simulink model "ISReferenceApplication"  (R2024b)
settings: Solver=ode4  StartTime=0.0  StopTime=60  FixedStep=1e-3  RelTol=5e-2
model workspace (MAT data in the model file):
  Downshift_Speeds = [9.5625  23.0625  36.5625  47.8125  59.0625  68.90625  78.75; 12.9375  26.4375  39.9375  51.1875  62.4375  72.84375  83.25; 16.3125  29.8125  43.3125  54.5625  65.8125  76.78125  87.75; 19.6875  33.1875  46.6875  57.9375  69.1875  80.71875  92.25]
  EngRevLim = 7000
  Pedal_Positions = [0.1 0.4 0.5 0.9]
  Upshift_Speeds = [12.9375  26.4375  39.9375  51.1875  62.4375  72.84375  83.25; 16.3125  29.8125  43.3125  54.5625  65.8125  76.78125  87.75; 19.6875  33.1875  46.6875  57.9375  69.1875  80.71875  92.25; 33  52.5  77.25  100.5  138.75  161.875  185]
  VEH.Mass = 1181
  VEH.StaticNormalFrontLoad.FR = 264.666666667
  VEH.StaticNormalFrontLoad.FL = 264.666666667
  VEH.StaticNormalRearLoad.RR = 322
  VEH.StaticNormalRearLoad.RL = 322
  VEH.WheelBase = 3.075
  VEH.FrontAxlePositionfromCG = 1.515
  VEH.RearAxlePositionfromCG = 1.504
  VEH.HeightCG = 0.134
  VEH.FrontalArea = 2.11
  VEH.DragCoefficient = 0.33
  VEH.NumberOfWheelsPerAxle = 2
  VEH.PitchMomentInertia = 1922.66666667
  VEH.RollMomentInertia = 432.333333333
  VEH.YawMomentInertia = 2066
  VEH.SteeringRatio = 18
  VEH.TrackWidth = 1.922
  VEH.SprungMass = 1096.72266667
  VEH.InitialLongPosition = 0
  VEH.InitialLatPosition = 0
  VEH.InitialVertPosition = 0
  VEH.InitialRollAngle = 0
  VEH.InitialPitchAngle = 0
  VEH.InitialYawAngle = 0
  VEH.InitialLongVel = 0
  VEH.InitialLatVel = 0
  VEH.InitialVertVel = 0
  VEH.InitialRollRate = 0
  VEH.InitialPitchRate = 0
  VEH.InitialYawRate = 0
  VEH.UnsprungMassRearAxle = 160
  VEH.UnsprungMassFrontAxle = 100
  rayDirections = [0  0  -1; 0  0  -1; 0  0  -1; 0  0  -1; 0  0  -1; 0  0  -1; 0  0  -1; 0  0  -1; 0  0  -1; 0  0  -1; 0  0  -1; 0  0  -1; 0  0  -1; 0  0  -1; 0  0  -1; 0  0  -1; 0  0  -1; 0  0  -1; 0  0  -1; 0  0  -1; 0  0  -1; 0  0  -1; 0  0  -1; 0  0  -1; 0  0  -1; 0  0  -1; 0  0  -1; 0  0  -1; 0  0  -1; 0  0  -1; 0  0  -1; 0  0  -1; 0  0  -1; 0  0  -1; 0  0  -1; 0  0  -1; 0  0  -1; 0  0  -1; 0  0  -1; 0  0  -1; 0  0  -1; 0  0  -1; 0  0  -1; 0  0  -1; 0  0  -1; 0  0  -1; 0  0  -1; 0  0  -1; 0  0  -1; 0  0  -1; 0  0  -1; 0  0  -1; 0  0  -1; 0  0  -1; 0  0  -1; 0  0  -1; 0  0  -1; 0  0  -1; 0  0  -1; 0  0  -1; 0  0  -1; 0  0  -1; 0  0  -1; 0  0  -1; 0  0  -1; 0  0  -1; 0  0  -1; 0  0  -1; 0  0  -1; 0  0  -1; 0  0  -1; 0  0  -1; 0  0  -1; 0  0  -1; 0  0  -1; 0  0  -1; 0  0  -1; 0  0  -1; 0  0  -1; 0  0  -1; 0  0  -1; 0  0  -1; 0  0  -1; 0  0  -1; 0  0  -1; 0  0  -1; 0  0  -1; 0  0  -1; 0  0  -1; 0  0  -1; 0  0  -1; 0  0  -1; 0  0  -1; 0  0  -1; 0  0  -1; 0  0  -1; 0  0  -1; 0  0  -1; 0  0  -1; 0  0  -1; 0  0  -1; 0  0  -1; 0  0  -1; 0  0  -1; 0  0  -1; 0  0  -1; 0  0  -1; 0  0  -1; 0  0  -1; 0  0  -1; 0  0  -1; 0  0  -1; 0  0  -1; 0  0  -1; 0  0  -1; 0  0  -1; 0  0  -1; 0  0  -1; 0  0  -1; 0  0  -1; 0  0  -1]
  rayLengths = [20; 20; 20; 20; 20; 20; 20; 20; 20; 20; 20; 20; 20; 20; 20; 20; 20; 20; 20; 20; 20; 20; 20; 20; 20; 20; 20; 20; 20; 20; 20; 20; 20; 20; 20; 20; 20; 20; 20; 20; 20; 20; 20; 20; 20; 20; 20; 20; 20; 20; 20; 20; 20; 20; 20; 20; 20; 20; 20; 20; 20; 20; 20; 20; 20; 20; 20; 20; 20; 20; 20; 20; 20; 20; 20; 20; 20; 20; 20; 20; 20; 20; 20; 20; 20; 20; 20; 20; 20; 20; 20; 20; 20; 20; 20; 20; 20; 20; 20; 20; 20; 20; 20; 20; 20; 20; 20; 20; 20; 20; 20; 20; 20; 20; 20; 20; 20; 20; 20; 20; 20]
  rayOrigins = [0.5  -0.5  0; 0.4  -0.5  0; 0.3  -0.5  0; 0.2  -0.5  0; 0.1  -0.5  0; 0  -0.5  0; -0.1  -0.5  0; -0.2  -0.5  0; -0.3  -0.5  0; -0.4  -0.5  0; -0.5  -0.5  0; 0.5  -0.4  0; 0.4  -0.4  0; 0.3  -0.4  0; 0.2  -0.4  0; 0.1  -0.4  0; 0  -0.4  0; -0.1  -0.4  0; -0.2  -0.4  0; -0.3  -0.4  0; -0.4  -0.4  0; -0.5  -0.4  0; 0.5  -0.3  0; 0.4  -0.3  0; 0.3  -0.3  0; 0.2  -0.3  0; 0.1  -0.3  0; 0  -0.3  0; -0.1  -0.3  0; -0.2  -0.3  0; -0.3  -0.3  0; -0.4  -0.3  0; -0.5  -0.3  0; 0.5  -0.2  0; 0.4  -0.2  0; 0.3  -0.2  0; 0.2  -0.2  0; 0.1  -0.2  0; 0  -0.2  0; -0.1  -0.2  0; -0.2  -0.2  0; -0.3  -0.2  0; -0.4  -0.2  0; -0.5  -0.2  0; 0.5  -0.1  0; 0.4  -0.1  0; 0.3  -0.1  0; 0.2  -0.1  0; 0.1  -0.1  0; 0  -0.1  0; -0.1  -0.1  0; -0.2  -0.1  0; -0.3  -0.1  0; -0.4  -0.1  0; -0.5  -0.1  0; 0.5  0  0; 0.4  0  0; 0.3  0  0; 0.2  0  0; 0.1  0  0; 0  0  0; -0.1  0  0; -0.2  0  0; -0.3  0  0; -0.4  0  0; -0.5  0  0; 0.5  0.1  0; 0.4  0.1  0; 0.3  0.1  0; 0.2  0.1  0; 0.1  0.1  0; 0  0.1  0; -0.1  0.1  0; -0.2  0.1  0; -0.3  0.1  0; -0.4  0.1  0; -0.5  0.1  0; 0.5  0.2  0; 0.4  0.2  0; 0.3  0.2  0; 0.2  0.2  0; 0.1  0.2  0; 0  0.2  0; -0.1  0.2  0; -0.2  0.2  0; -0.3  0.2  0; -0.4  0.2  0; -0.5  0.2  0; 0.5  0.3  0; 0.4  0.3  0; 0.3  0.3  0; 0.2  0.3  0; 0.1  0.3  0; 0  0.3  0; -0.1  0.3  0; -0.2  0.3  0; -0.3  0.3  0; -0.4  0.3  0; -0.5  0.3  0; 0.5  0.4  0; 0.4  0.4  0; 0.3  0.4  0; 0.2  0.4  0; 0.1  0.4  0; 0  0.4  0; -0.1  0.4  0; -0.2  0.4  0; -0.3  0.4  0; -0.4  0.4  0; -0.5  0.4  0; 0.5  0.5  0; 0.4  0.5  0; 0.3  0.5  0; 0.2  0.5  0; 0.1  0.5  0; 0  0.5  0; -0.1  0.5  0; -0.2  0.5  0; -0.3  0.5  0; -0.4  0.5  0; -0.5  0.5  0]
  temp.Mass = 1181
  temp.StaticNormalFrontLoad.FR = 264.666666667
  temp.StaticNormalFrontLoad.FL = 264.666666667
  temp.StaticNormalRearLoad.RR = 322
  temp.StaticNormalRearLoad.RL = 322
  temp.WheelBase = 2.86
  temp.FrontAxlePositionfromCG = 1.43
  temp.RearAxlePositionfromCG = 1.43
  temp.HeightCG = 0.134
  temp.FrontalArea = 2.11
  temp.DragCoefficient = 0.33
  temp.NumberOfWheelsPerAxle = 2
  temp.PitchMomentInertia = 1922.66666667
  temp.RollMomentInertia = 432.333333333
  temp.YawMomentInertia = 2066
  temp.SteeringRatio = 18
  temp.TrackWidth = 1.485
  temp.SprungMass = 1096.72266667
  temp.InitialLongPosition = 590.01904884
  temp.InitialLatPosition = 11.2130507532
  temp.InitialVertPosition = -0.6630556109
  temp.InitialRollAngle = -0.0172848662
  temp.InitialPitchAngle = 0.0033932423
  temp.InitialYawAngle = 0.001924738
  temp.InitialLongVel = 0
  temp.InitialLatVel = 0
  temp.InitialVertVel = 0
  temp.InitialRollRate = 0
  temp.InitialPitchRate = 0
  temp.InitialYawRate = 0
  temp.UnsprungMassRearAxle = 160
  temp.UnsprungMassFrontAxle = 100
  temp.VehicleWidth = 1.731
  temp.VehicleLength = 4.769
  temp.diameter = 0.653
  temp.DrawFreq = 0.1
  temp.T_ref = [0 0.173579329608 0.347158660043 0.520737996807 0.69431733453 0.867896671781 1.04147600843 1.21505534588 1.38863468425 1.56221402051 1.73579335734 1.90937269505 ... (14403 elements, 4801x3)]
undefined symbols (not defined in the file): DiscIntNeverNeededParam, Sim3dSensor
libraries: simulink x14, autolibutils x7, slpidlib x2, vehdynlibviscommon x2, sim3dgroundtruthsensorlib x2, autolibtranscontrolscommon x1, autolibshared x1, vehdynlibdriver x1, sharedtransform x1, vehdynlibsens x1, vehdynlibscenariocommon x1, sim3dlib x1
(part 1 of 4)
settings Model: DataDictionary=ISReferenceApplication.sldd  ModifiedByFormat=The MathWorks, Inc.  SimulationMode=accelerator  Creator=The MathWorks, Inc.  LastModifiedBy=The MathWorks, Inc.
settings SolverCC: SolverJacobianMethodControl=FullPerturbation  ZeroCrossAlgorithm=Adaptive  AlgebraicLoopSolver=TrustRegion  DecoupledContinuousIntegration=on  MinimalZcImpactIntegration=on  MaxZcPerStep=1
settings DataIOCC: ReturnWorkspaceOutputs=off
settings OptimizationCC: ReuseModelBlockBuffer=off
settings DebuggingCC: SignalInfNanChecking=error  ArtificialAlgebraicLoopMsg=none  MaskedZcDiagnostic=none  IgnoredZcDiagnostic=none  UnconnectedInputMsg=warning  UnconnectedOutputMsg=warning  UnconnectedLineMsg=warning  PregeneratedLibrarySubsystemCodeDiagnostic=none  ArithmeticOperatorsInVariantConditions=warning
settings ModelReferenceCC: UpdateModelReferenceTargets=IfOutOfDate  EnableRefExpFcnMdlSchedulingChecks=on  ModelReferenceMinAlgLoopOccurrences=on  PropagateSignalLabelsOutOfModel=off
settings SFSimCC: SimUseLocalCustomCode=off
settings RTWCC: RTWUseLocalCustomCode=off  GPUComputeCapability=3.5  DLArmComputeVersion=19.05

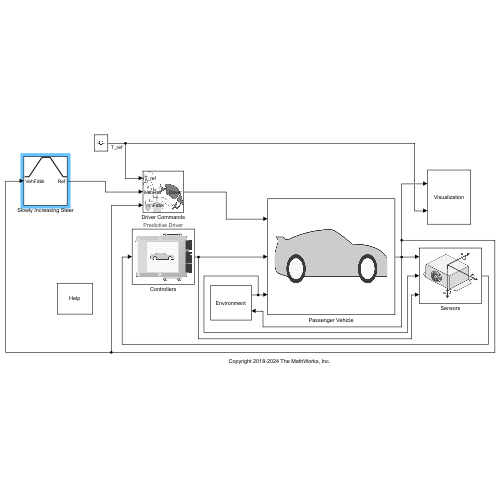
[thumbnail: Simulink's stored preview of the top-level diagram]
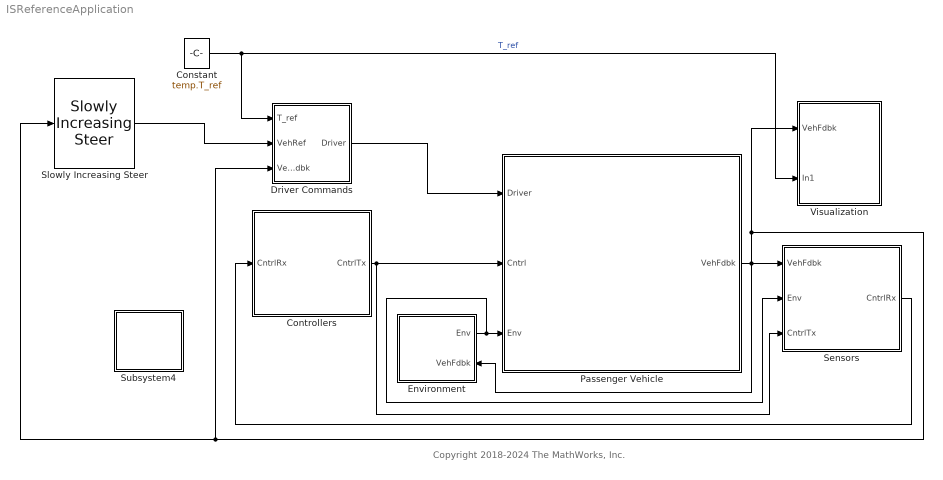
== system ISReferenceApplication ==
  note: Copyright 2018-2024 The MathWorks, Inc.
  Constant : Constant  Value=temp.T_ref  VectorParams1D=off
  Controllers : Subsystem
      mask Display: image('SystemControllers.png')
  Driver Commands : Subsystem  VariantControl=0  mask{driverType=Predictive Driver}
      mask prompts: driverType "Vehicle command mode"
      mask init:
      | [~]=vdynblksdrvrconfig(gcb)
      settings: AttributesFormatString=%<driverType>
      mask Help: eval('vdynblkshelp(''vdcrdriver'')');
      mask TypeOptions driverType: Longitudinal Driver | Predictive Driver | Open Loop
      mask Display: image('driverlatlong.png');
  Environment : Subsystem
      settings: PortSchema="{\"entries\":[{\"content\":{\"sides\":[{\"content\":{\"connectorIds\":[]},\"type\":\"ConnectorPlacement.EquallySpacedRectSide\",\"uuid\":\"7e477c5b-2979-4b31-83f8-8e06b5171f31\"},{\"content\":{\"connectorIds\":[\"Out1\",\"In1\"],\"side\":\"RIGHT\"},\"type\":\"ConnectorPlacement.EquallySpacedRectSide\",\"uuid\":\"d70ab29f-7073-466b-949c-fd6d019fdbd7\"},{\"content\":{\"connectorIds\":[],\"side\":\"TOP\"},\"type\":\"ConnectorPlacement.EquallySpacedRectSide\",\"uuid\":\"2d86cca8-a415-4272-bacd-17a50325dd7c\"}]},\"type\":\"ConnectorPlacement.EquallySpacedConnector\",\"uuid\":\"3f48fc9c-531e-41c0-b546-1206e5799aa8\"}],\"packageUris\":[\"http://schema.mathworks.com/mf0/Connector/R2020b\"],\"version\":\"1.0\"}"
      mask Display: disp('Environment')
  Passenger Vehicle : Subsystem
      mask Display: image('PassengerVehicle.png')
  Sensors : Subsystem
      mask Display: image('sensorimu.png'); % Use "Edit Image" on toolstrip to change.
  Slowly Increasing Steer : vehdynlibscenariocommon/Slowly Increasing Steer  ssMode=Initialize from model  ssVar=logsout  t_start=0  xdot_r=40  xdotUnit=km/hr  omega_hw=10  theta_max=270  t_stop=2  ay_max=.5  steerDir=off  ay_stop=off  ssDefault=on  X_o=0  Y_o=0  psi_o=0  ssTol=0.0001  ssMaxTime=10  ssWSName=is50mph  aMode=2
  Subsystem4 : Subsystem
      settings: OpenFcn=eval('vdynblkshelp(''vdynblksincreasingsteering'')');
      mask Display: disp('Help')
  Visualization : Subsystem
      mask Display: disp('Visualization')
  wires:
  Controllers/1(CntrlTx) -> Sensors/3(CntrlTx), Passenger Vehicle/2(Cntrl)
  Slowly Increasing Steer/1 -> Driver Commands/2(VehRef)
  Driver Commands/1(Driver) -> Passenger Vehicle/1(Driver)
  Sensors/1(CntrlRx) -> Controllers/1(CntrlRx)
  Environment/1(Env) -> Passenger Vehicle/3(Env), Sensors/2(Env)
  Passenger Vehicle/1(VehFdbk) -> Environment/1(VehFdbk), Sensors/1(VehFdbk), Visualization/1(VehFdbk), Driver Commands/3(VehFdbk), Slowly Increasing Steer/1
  Constant/1 -> Driver Commands/1(T_ref), Visualization/2(In1)  "T_ref"

== system ISReferenceApplication/Controllers ==
  CntrlRx : Inport
  Active Differential Control : Subsystem  Variant=on  VariantControlMode=label  LabelModeActiveChoice=0
  Brake Pressure Control : Subsystem  Variant=on  VariantControlMode=label  LabelModeActiveChoice=0
  Bus Creator : BusCreator  Inputs=1
  Bus Creator1 : BusCreator  Inputs=1
  Bus Creator2 : BusCreator  Inputs=3
  Bus Creator3 : BusCreator  Inputs=4
  Bus Creator4 : BusCreator  Inputs=1
  Bus Selector : BusSelector  OutputSignals=Driver.DecelFdbk,Wheels.Omega,IMU.Acc,Driver.AccFdbk,Wheels.BrkPrs
  Bus Selector1 : BusSelector  OutputSignals=Driver.AccFdbk,Driver.DecelFdbk,Driver.GearFdbk,Engine.EngSpd,Wheels.Omega
  Bus Selector2 : BusSelector  OutputSignals=Driver.AccFdbk,Engine.EngSpd
  Bus Selector3 : BusSelector  OutputSignals=Driver.AccFdbk,Driver.DecelFdbk,Driver.SteerFdbk,Driver.GearFdbk,Wheels.Omega,IMU.Acc,IMU.pqr
  ECU : Subsystem  SystemSampleTime=.01
  Ground : Ground
  Transmission Controller : Subsystem  Variant=on  VariantControlMode=label  VariantControl=Variant1  LabelModeActiveChoice=3
  CntrlTx : Outport  VectorParamsAs1DForOutWhenUnconnected=off
  wires:
  Bus Selector2/1 -> ECU/2(<Accel>)  "<AccFdbk>"
  Bus Creator/1 -> Bus Creator3/1  "ECU"
  Bus Creator1/1 -> Bus Creator3/2  "Transmission"
  Bus Creator3/1 -> CntrlTx/1  "CntrlTx"
  Bus Creator4/1 -> Bus Creator3/4  "Diff"
  Active Differential Control/1(DiffPrsCmd) -> Bus Creator4/1  "DiffPrsCmd"
  Active Differential Control/2(TrqCmd) -> [DiffTrqCmd]
  ECU/1(EngTrqCmd) -> Bus Creator/1  "EngTrqCmd"
  Transmission Controller/1(" Gear") -> Bus Creator1/1  "GearCmd"
  [DiffTrqCmd] -> ECU/1(DiffTrqCmd)  "DiffTrqCmd"
  Ground/1 -> Transmission Controller/7(UpReq), Transmission Controller/8(DownReq)
  Bus Selector2/2 -> ECU/3(EngSpd)  "<EngSpd>"
  Bus Selector1/5 -> Transmission Controller/5(Omega)  "<Omega>"
  Bus Selector1/2 -> Transmission Controller/2(BrkCmd)  "<DecelFdbk>"
  Bus Selector1/3 -> Transmission Controller/3(GearReq)  "<GearFdbk>"
  Bus Selector1/4 -> Transmission Controller/4(EngSpd)  "<EngSpd>"
  Bus Selector1/1 -> Transmission Controller/1(Accel)  "<AccFdbk>"
  Bus Selector3/1 -> Active Differential Control/1(Accel)  "<AccFdbk>"
  Bus Selector3/2 -> Active Differential Control/2(BrkCmd)  "<DecelFdbk>"
  Bus Selector3/3 -> Active Differential Control/3(Steer)  "<SteerFdbk>"
  Bus Selector3/4 -> Active Differential Control/4(GearFdbk)  "<GearFdbk>"
  Bus Selector3/5 -> Active Differential Control/5(Omega)  "<Omega>"
  Bus Selector3/6 -> Active Differential Control/6(axayaz)  "<Acc>"
  Bus Selector3/7 -> Active Differential Control/7(pqr)  "<pqr>"
  Bus Selector/1 -> Brake Pressure Control/1(DecelFdbk)  "<DecelFdbk>"
  CntrlRx/1 -> Bus Selector3/1, Bus Selector/1, Bus Selector1/1, Bus Selector2/1
  Bus Selector/2 -> Brake Pressure Control/2(Omega)  "<Omega>"
  Bus Selector/3 -> Brake Pressure Control/3(Accel)  "<Acc>"
  Brake Pressure Control/2(BrkPrsCmd) -> Bus Creator2/2  "BrkPrsCmd"
  Bus Creator2/1 -> Bus Creator3/3  "Brake"
  Brake Pressure Control/1(ABSFlag) -> [ABSFlag], Bus Creator2/1  "ABSFlag"
  [ABSFlag] -> Transmission Controller/6(ABSFlag)
  [ABSFlag] -> ECU/4(ABSFlag)
  Bus Selector/4 -> Brake Pressure Control/4(AccelFdbk)  "<AccFdbk>"
  Bus Selector/5 -> Brake Pressure Control/5(BrkPrs)  "<BrkPrs>"
  Brake Pressure Control/3(TCSFlag) -> Bus Creator2/3  "TCSFlag"

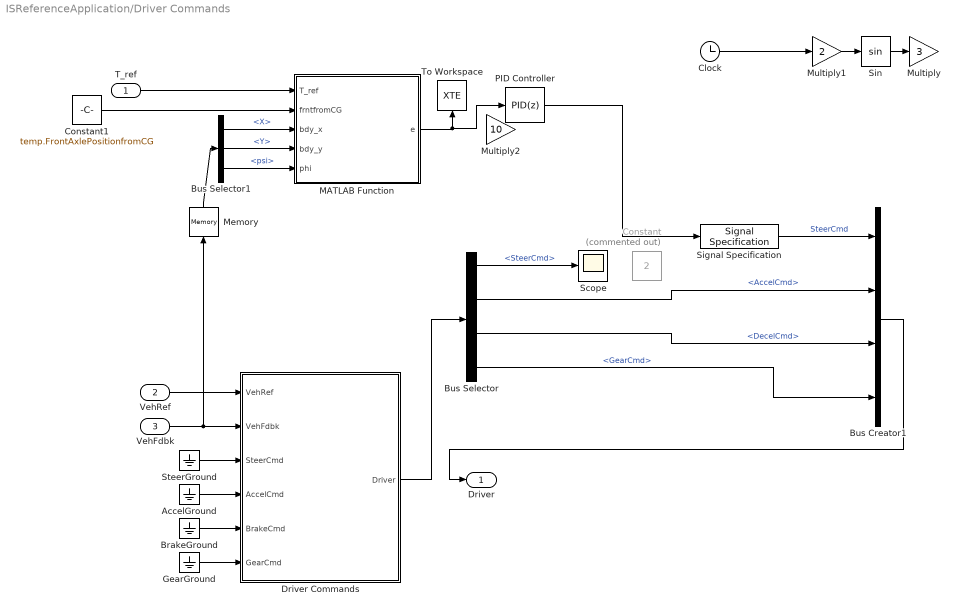
== system ISReferenceApplication/Driver Commands ==
  T_ref : Inport
  VehRef : Inport  Port=2
  VehFdbk : Inport  Port=3
  AccelGround : Ground
  BrakeGround : Ground
  Bus Creator1 : BusCreator  Inputs=4
  Bus Selector : BusSelector  OutputSignals=SteerCmd,AccelCmd,DecelCmd,GearCmd
  Bus Selector1 : BusSelector  OutputSignals=Body.InertFrm.Geom.Disp.X,Body.InertFrm.Geom.Disp.Y,Body.InertFrm.Cg.Ang.psi
  Clock : Clock
  Constant : Constant  Commented=on  Value=2
  Constant1 : Constant  Value=temp.FrontAxlePositionfromCG
  Driver Commands : Subsystem  Variant=on  VariantControl=Variant1  AllowZeroVariantControls=on
  GearGround : Ground
  MATLAB Function : MATLAB Function  TreatAsAtomicUnit=on
  Memory : Memory
  Multiply : Gain  Gain=3
  Multiply1 : Gain  Gain=2
  Multiply2 : Gain  Gain=10
  PID Controller : slpidlib/PID Controller  Controller=PID  Form=Parallel  TimeDomain=Discrete-time  UseExternalTs=off  SampleTime=-1  IntegratorMethod=Forward Euler  FilterMethod=Forward Euler  ControllerParametersSource=internal  P=10  I=10  UseKiTs=off  D=5  UseExternalDerivativeSource=off  N=100  UseFilter=on  TunerSelectOption=Transfer Function Based (PID Tuner App)  InitialConditionSource=internal  InitialConditionForIntegrator=0  InitialConditionForFilter=0  DifferentiatorICPrevScaledInput=0  ExternalReset=none  TrackingMode=off  Kt=1  LimitOutput=off  SatLimitsSource=internal  UpperSaturationLimit=inf  LowerSaturationLimit=-inf  LinearizeAsGain=on  AntiWindupMode=none  Kb=1  LimitIntegrator=off  UpperIntegratorSaturationLimit=inf  LowerIntegratorSaturationLimit=-inf  POutMin=[]  POutMax=[]  IOutMin=[]  IOutMax=[]  DOutMin=[]  DOutMax=[]  NOutMin=[]  NOutMax=[]  SumOutMin=[]  SumOutMax=[]  SaturationOutMin=[]  SaturationOutMax=[]  PParamMin=[]  PParamMax=[]  IParamMin=[]  IParamMax=[]  DParamMin=[]  DParamMax=[]  NParamMin=[]  NParamMax=[]  KbParamMin=[]  KbParamMax=[]  KtParamMin=[]  KtParamMax=[]  KbOutMin=[]  KbOutMax=[]  KtOutMin=[]  KtOutMax=[]  IntegratorOutMin=[]  IntegratorOutMax=[]  FilterOutMin=[]  FilterOutMax=[]  SumI1OutMin=[]  SumI1OutMax=[]  SumI2OutMin=[]  SumI2OutMax=[]  SumI3OutMin=[]  SumI3OutMax=[]  SumI4OutMin=[]  SumI4OutMax=[]  SumDOutMin=[]  SumDOutMax=[]  DifferentiatorOutMin=[]  DifferentiatorOutMax=[]  FilterDiffOutCoefMin=[]  FilterDiffOutCoefMax=[]  ReciprocalOutMin=[]  ReciprocalOutMax=[]  SumDenOutMin=[]  SumDenOutMax=[]  SumNumOutMin=[]  SumNumOutMax=[]  DivideOutMin=[]  DivideOutMax=[]  UdiffTsProdOutMin=[]  UdiffTsProdOutMax=[]  NTsProdOutMin=[]  NTsProdOutMax=[]  UintegralTsProdOutMin=[]  UintegralTsProdOutMax=[]  UngainTsProdOutMin=[]  UngainTsProdOutMax=[]  ClampingZeroOutDataTypeStr=Inherit: Inherit via back propagation  ClampingZeroOutMin=[]  ClampingZeroOutMax=[]  FilterDenConstantOutDataTypeStr=Inherit: Inherit via back propagation  FilterDenConstantOutMin=[]  FilterDenConstantOutMax=[]  PCopyOutDataTypeStr=Inherit: Inherit via back propagation  PCopyOutMin=[]  PCopyOutMax=[]  NCopyOutDataTypeStr=Inherit: Inherit via back propagation  NCopyOutMin=[]  NCopyOutMax=[]  IntegratorContinuousStateAttributes=''  IntegratorStateMustResolveToSignalObject=off  IntegratorRTWStateStorageClass=Auto  FilterContinuousStateAttributes=''  FilterStateMustResolveToSignalObject=off  FilterRTWStateStorageClass=Auto  ParallelPVariant=InternalParameters  IdealPVariant=Disabled  IVariant=InternalParameters  DVariant=InternalParameters  IntegratorVariant=Discrete  SatVariant=Disabled  AWVariant=Passthrough  PCopyVariant=Disabled  TRVariant=Disabled  FdbkBlocksVariant=Forward  IdealPFdbkVariant=Disabled  SatFdbkVariant=Disabled  DerivativeFilterVariant=ForwardEulerFilter  NVariant=InternalParameters  NCopyVariant=Disabled  FilterICVariant=InternalICsFilter  IntegratorICVariant=InternalICs  ExternalResetVariant=Disabled  TRSumVariant=Passthrough  SumFdbkVariant=Disabled  SumVariant=Sum_PID  TsampFilterVariant=InternalTs  TsampNgainVariant=Passthrough  TsampIntegralVariant=Disabled_SignalSpec  ExternalSaturationOutDataTypeStr=Inherit: Same as second input  DerivativeSourceVariant=ErrorSignal  PreIntVariant=InternalPreInt
  Scope : Scope
  Signal Specification : SignalSpecification  Unit=rad
  Sin : Trigonometry
  SteerGround : Ground
  To Workspace : ToWorkspace  VariableName=XTE  SaveFormat=Timeseries  SampleTime=-1
  Driver : Outport  VectorParamsAs1DForOutWhenUnconnected=off
  wires:
  VehRef/1 -> Driver Commands/1(VehRef)
  VehFdbk/1 -> Memory/1, Driver Commands/2(VehFdbk)
  Driver Commands/1(" Driver") -> Bus Selector/1
  SteerGround/1 -> Driver Commands/3(SteerCmd)
  AccelGround/1 -> Driver Commands/4(AccelCmd)
  BrakeGround/1 -> Driver Commands/5(BrakeCmd)
  GearGround/1 -> Driver Commands/6(GearCmd)
  Bus Selector/2 -> Bus Creator1/2  "<AccelCmd>"
  Bus Selector/3 -> Bus Creator1/3  "<DecelCmd>"
  Bus Selector/4 -> Bus Creator1/4  "<GearCmd>"
  Bus Selector/1 -> Scope/1  "<SteerCmd>"
  Signal Specification/1 -> Bus Creator1/1  "SteerCmd"
  Bus Creator1/1 -> Driver/1
  Clock/1 -> Multiply1/1
  Sin/1 -> Multiply/1
  Multiply1/1 -> Sin/1
  T_ref/1 -> MATLAB Function/1(T_ref)
  Bus Selector1/1 -> MATLAB Function/3(bdy_x)  "<X>"
  Bus Selector1/2 -> MATLAB Function/4(bdy_y)  "<Y>"
  Bus Selector1/3 -> MATLAB Function/5(phi)  "<psi>"
  MATLAB Function/1(e) -> PID Controller/1, To Workspace/1
  Memory/1 -> Bus Selector1/1
  Constant1/1 -> MATLAB Function/2(frntfromCG)
  PID Controller/1 -> Signal Specification/1

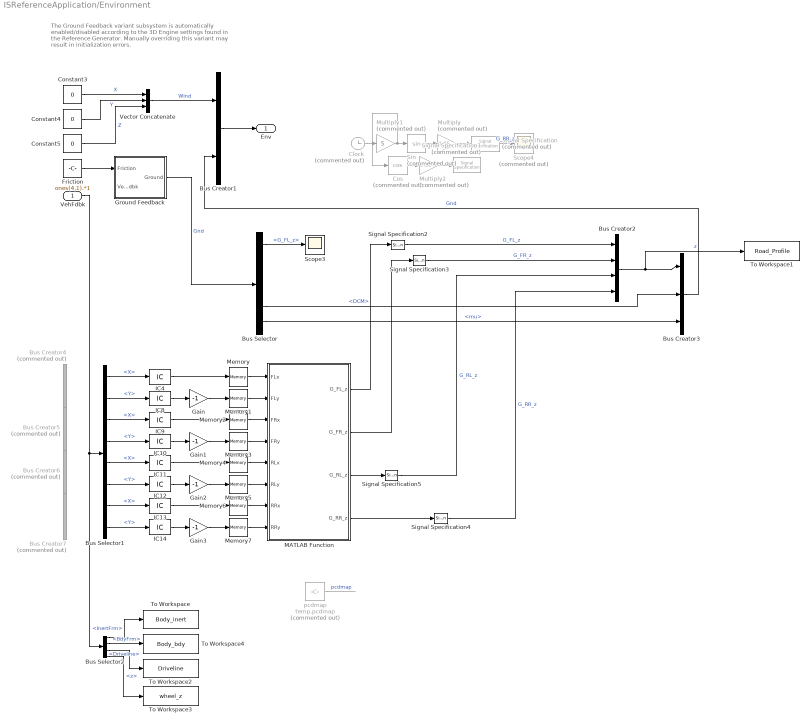
== system ISReferenceApplication/Environment ==
  note: The Ground Feedback variant subsystem is automatically enabled/disabled according to the 3D Engine settings found in the Reference Generator.
      | Manually overriding this variant may result in initialization errors.
  VehFdbk : Inport
  Bus Creator1 : BusCreator  Inputs=2
  Bus Creator2 : BusCreator  Inputs=4
  Bus Creator3 : BusCreator  Inputs=3
  Bus Creator{4..7} (4 alike) : BusCreator  Commented=on  Inputs=2
  Bus Selector : BusSelector  OutputSignals=z.G_FL_z,z.G_FR_z,z.G_RL_z,z.G_RR_z,DCM,mu
  Bus Selector1 : BusSelector  OutputSignals=Body.InertFrm.FrntAxl.Lft.Disp.X,Body.InertFrm.FrntAxl.Lft.Disp.Y,Body.InertFrm.FrntAxl.Rght.Disp.X,Body.InertFrm.FrntAxl.Rght.Disp.Y,Body.InertFrm.RearAxl.Lft.Disp.X,Body.InertFrm.RearAxl.Lft.Disp.Y,Body.InertFrm.RearAxl.Rght.Disp.X,Body.InertFrm.RearAxl.Rght.Disp.Y
  Bus Selector2 : BusSelector  OutputSignals=Body.InertFrm,Body.BdyFrm,Driveline,Wheels.TireFrame.z
  Clock : Clock  Commented=on
  Constant3 : Constant  Value=0
  Constant4 : Constant  Value=0
  Constant5 : Constant  Value=0
  Cos : Trigonometry  Commented=on  Operator=cos
  Friction : Constant  Value=ones(4,1).*1
  Gain{,1..3} (4 alike) : Gain  Gain=-1
  Ground Feedback : Subsystem  Variant=on  VariantControlMode=label  LabelModeActiveChoice=0
  IC{4,8..14} (8 alike) : InitialCondition  Value=0
  MATLAB Function : MATLAB Function  TreatAsAtomicUnit=on
  Memory : Memory  InitialCondition=temp.InitialLongPosition+temp.FrontAxlePositionfromCG  InheritSampleTime=on
  Memory1 : Memory  InitialCondition=-temp.InitialLatPosition-temp.TrackWidth  InheritSampleTime=on
  Memory2 : Memory  InitialCondition=temp.InitialLongPosition+temp.FrontAxlePositionfromCG  InheritSampleTime=on
  Memory3 : Memory  InitialCondition=-temp.InitialLatPosition+temp.TrackWidth  InheritSampleTime=on
  Memory4 : Memory  InitialCondition=temp.InitialLongPosition+temp.RearAxlePositionfromCG  InheritSampleTime=on
  Memory5 : Memory  InitialCondition=-temp.InitialLatPosition-temp.TrackWidth  InheritSampleTime=on
  Memory6 : Memory  InitialCondition=temp.InitialLongPosition+temp.RearAxlePositionfromCG  InheritSampleTime=on
  Memory7 : Memory  InitialCondition=-temp.InitialLatPosition+temp.TrackWidth  InheritSampleTime=on
  Multiply : Gain  Commented=on  Gain=0.05
  Multiply1 : Gain  Commented=on  Gain=5
  Multiply2 : Gain  Commented=on  Gain=0.05
  Scope3 : Scope
  Scope4 : Scope  Commented=on
  Signal Specification : SignalSpecification  Commented=on  Unit=m
  Signal Specification1 : SignalSpecification  Commented=on  Unit=m
  Signal Specification{2..5} (4 alike) : SignalSpecification  OutDataTypeStr=double  Unit=m
  Sin : Trigonometry  Commented=on
  To Workspace : ToWorkspace  VariableName=Body_inert  SaveFormat=Timeseries  SampleTime=-1
  To Workspace1 : ToWorkspace  VariableName=Road_Profile  SaveFormat=Timeseries  SampleTime=-1
  To Workspace2 : ToWorkspace  VariableName=Driveline  SaveFormat=Timeseries  SampleTime=-1
  To Workspace3 : ToWorkspace  VariableName=wheel_z  SaveFormat=Timeseries  SampleTime=-1
  To Workspace4 : ToWorkspace  VariableName=Body_bdy  SaveFormat=Timeseries  SampleTime=-1
  Vector Concatenate : Concatenate  NumInputs=3
  pcdmap : Constant  Commented=on  Value=temp.pcdmap
  Env : Outport  VectorParamsAs1DForOutWhenUnconnected=off
  wires:
  Constant5/1 -> Vector Concatenate/3  "Z"
  Vector Concatenate/1 -> Bus Creator1/1  "Wind"
  Constant3/1 -> Vector Concatenate/1  "X"
  Constant4/1 -> Vector Concatenate/2  "Y"
  Bus Creator1/1 -> Env/1
  Friction/1 -> Ground Feedback/1(Friction)
  VehFdbk/1 -> Bus Selector2/1, Bus Selector1/1
  Sin/1 -> Multiply/1
  Multiply/1 -> Signal Specification/1
  Signal Specification/1 -> Scope4/1  "G_RR_z"
  Bus Creator2/1 -> To Workspace1/1, Bus Creator3/1  "z"
  Bus Selector/5 -> Bus Creator3/2  "<DCM>"
  Bus Selector/6 -> Bus Creator3/3  "<mu>"
  Clock/1 -> Multiply1/1
  Multiply1/1 -> Cos/1, Sin/1
  Multiply2/1 -> Signal Specification1/1
  Cos/1 -> Multiply2/1
  Bus Selector/1 -> Scope3/1  "<G_FL_z>"
  pcdmap/1 -> ?  "pcdmap"
  Bus Selector1/1 -> IC4/1  "<X>"
  Bus Selector1/2 -> IC8/1  "<Y>"
  Bus Selector1/3 -> IC9/1  "<X>"
  Bus Selector1/4 -> IC10/1  "<Y>"
  Bus Selector1/5 -> IC11/1  "<X>"
  Bus Selector1/6 -> IC12/1  "<Y>"
  Bus Selector1/7 -> IC13/1  "<X>"
  Bus Selector1/8 -> IC14/1  "<Y>"
  IC4/1 -> Memory/1
  IC8/1 -> Gain/1
  IC9/1 -> Memory2/1
  IC10/1 -> Gain1/1
  IC11/1 -> Memory4/1
  IC12/1 -> Gain2/1
  IC13/1 -> Memory6/1
  IC14/1 -> Gain3/1
  Signal Specification2/1 -> Bus Creator2/1  "G_FL_z"
  Signal Specification3/1 -> Bus Creator2/2  "G_FR_z"
  Signal Specification4/1 -> Bus Creator2/4  "G_RR_z"
  Signal Specification5/1 -> Bus Creator2/3  "G_RL_z"
  MATLAB Function/1(G_FL_z) -> Signal Specification2/1
  MATLAB Function/2(G_FR_z) -> Signal Specification3/1
  MATLAB Function/3(G_RL_z) -> Signal Specification5/1
  MATLAB Function/4(G_RR_z) -> Signal Specification4/1
  Memory/1 -> MATLAB Function/1(FLx)
  Memory1/1 -> MATLAB Function/2(FLy)
  Memory2/1 -> MATLAB Function/3(FRx)
  Memory3/1 -> MATLAB Function/4(FRy)
  Memory4/1 -> MATLAB Function/5(RLx)
  Memory5/1 -> MATLAB Function/6(RLy)
  Memory6/1 -> MATLAB Function/7(RRx)
  Memory7/1 -> MATLAB Function/8(RRy)
  Gain/1 -> Memory1/1
  Gain1/1 -> Memory3/1
  Gain2/1 -> Memory5/1
  Gain3/1 -> Memory7/1
  Bus Selector2/1 -> To Workspace/1  "<InertFrm>"
  Bus Selector2/3 -> To Workspace2/1  "<Driveline>"
  Ground Feedback/1(Ground) -> Bus Selector/1  "Gnd"
  Bus Creator3/1 -> Bus Creator1/2  "Gnd"
  Bus Selector2/4 -> To Workspace3/1  "<z>"
  Bus Selector2/2 -> To Workspace4/1  "<BdyFrm>"

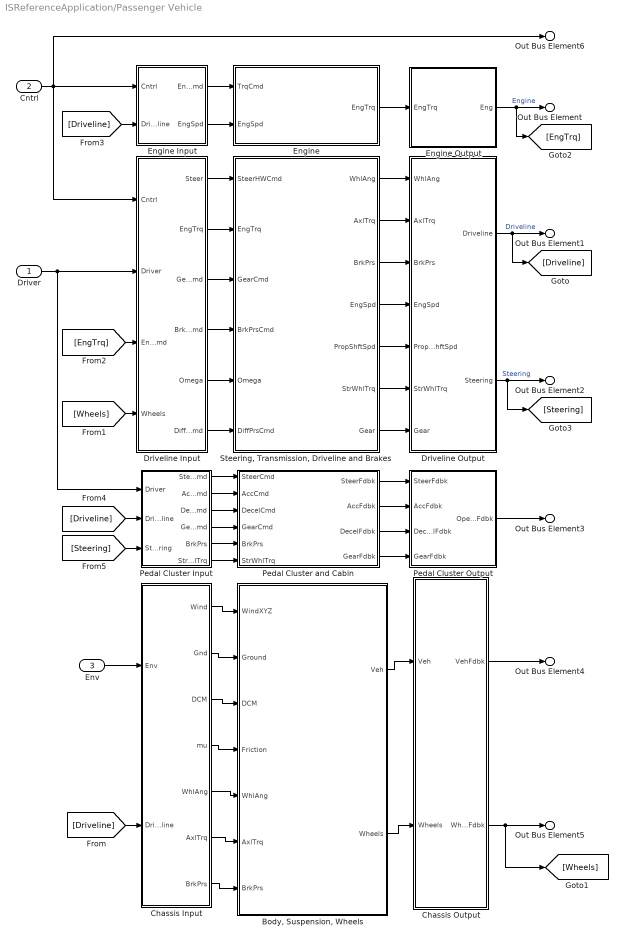
== system ISReferenceApplication/Passenger Vehicle ==
  Driver : Inport
  Cntrl : Inport  Port=2
  Env : Inport  Port=3
  "Body, Suspension, Wheels" : Subsystem  Variant=on  VariantControlMode=label  LabelModeActiveChoice=3
  Chassis Input : Subsystem
  Chassis Output : Subsystem
  Driveline Input : Subsystem
  Driveline Output : Subsystem
  Engine : Subsystem  Variant=on  VariantControlMode=label  LabelModeActiveChoice=0
  Engine Input : Subsystem
  Engine Output : Subsystem
  Pedal Cluster Input : Subsystem
  Pedal Cluster Output : Subsystem
  Pedal Cluster and Cabin : Subsystem
  "Steering, Transmission, Driveline and Brakes" : Subsystem  Variant=on  VariantControlMode=label  LabelModeActiveChoice=0
  Out Bus Element : Outport  PortName=VehFdbk  Element=Engine
  Out Bus Element1 : Outport  PortName=VehFdbk  Element=Driveline
  Out Bus Element2 : Outport  PortName=VehFdbk  Element=Steering
  Out Bus Element3 : Outport  PortName=VehFdbk  Element=Driver
  Out Bus Element4 : Outport  PortName=VehFdbk  Element=Body
  Out Bus Element5 : Outport  PortName=VehFdbk  Element=Wheels
  Out Bus Element6 : Outport  PortName=VehFdbk  Element=Cntrl
  wires:
  Env/1 -> Chassis Input/1(Env)
  Chassis Input/1(Wind) -> "Body, Suspension, Wheels"/1(WindXYZ)
  Chassis Input/2(Gnd) -> "Body, Suspension, Wheels"/2(Ground)
  Chassis Input/4(mu) -> "Body, Suspension, Wheels"/4(Friction)
  Chassis Input/5(WhlAng) -> "Body, Suspension, Wheels"/5(WhlAng)
  Chassis Input/6(AxlTrq) -> "Body, Suspension, Wheels"/6(AxlTrq)
  Chassis Input/7(BrkPrs) -> "Body, Suspension, Wheels"/7(BrkPrs)
  Driveline Output/1(Driveline) -> Out Bus Element1/1, [Driveline]  "Driveline"
  "Steering, Transmission, Driveline and Brakes"/1(WhlAng) -> Driveline Output/1(WhlAng)
  "Steering, Transmission, Driveline and Brakes"/2(AxlTrq) -> Driveline Output/2(AxlTrq)
  "Steering, Transmission, Driveline and Brakes"/3(BrkPrs) -> Driveline Output/3(BrkPrs)
  "Steering, Transmission, Driveline and Brakes"/4(EngSpd) -> Driveline Output/4(EngSpd)
  "Steering, Transmission, Driveline and Brakes"/5(PropShftSpd) -> Driveline Output/5(PropShftSpd)
  Driver/1 -> Pedal Cluster Input/1(Driver), Driveline Input/2(Driver)
  Cntrl/1 -> Out Bus Element6/1, Engine Input/1(Cntrl), Driveline Input/1(Cntrl)
  Driveline Input/1(Steer) -> "Steering, Transmission, Driveline and Brakes"/1(SteerHWCmd)
  Driveline Input/3(GearCmd) -> "Steering, Transmission, Driveline and Brakes"/3(GearCmd)
  Driveline Input/4(BrkPrsCmd) -> "Steering, Transmission, Driveline and Brakes"/4(BrkPrsCmd)
  Driveline Input/5(Omega) -> "Steering, Transmission, Driveline and Brakes"/5(Omega)
  Engine/1(EngTrq) -> Engine Output/1("EngTrq ")
  Driveline Input/2(EngTrq) -> "Steering, Transmission, Driveline and Brakes"/2(EngTrq)
  Engine Input/1(EngTrqCmd) -> Engine/1(TrqCmd)
  Engine Input/2(EngSpd) -> Engine/2(EngSpd)
  Engine Output/1(Eng) -> Out Bus Element/1, [EngTrq]  "Engine"
  [Driveline] -> Chassis Input/2(Driveline)
  [Wheels] -> Driveline Input/4(Wheels)
  [EngTrq] -> Driveline Input/3(EngTrqCmd)
  [Driveline] -> Engine Input/2(Driveline)
  Driveline Input/6(DiffPrsCmd) -> "Steering, Transmission, Driveline and Brakes"/6(DiffPrsCmd)
  "Steering, Transmission, Driveline and Brakes"/6(StrWhlTrq) -> Driveline Output/6(StrWhlTrq)
  Driveline Output/2(Steering) -> Out Bus Element2/1, [Steering]  "Steering"
  Pedal Cluster Output/1(OperatorFdbk) -> Out Bus Element3/1
  Pedal Cluster and Cabin/1(SteerFdbk) -> Pedal Cluster Output/1(SteerFdbk)
  Pedal Cluster and Cabin/2(AccFdbk) -> Pedal Cluster Output/2(AccFdbk)
  Pedal Cluster and Cabin/3(DecelFdbk) -> Pedal Cluster Output/3(DecelFdbk)
  Pedal Cluster and Cabin/4(GearFdbk) -> Pedal Cluster Output/4(GearFdbk)
  Pedal Cluster Input/4(GearCmd) -> Pedal Cluster and Cabin/4(GearCmd)
  Pedal Cluster Input/3(DecelCmd) -> Pedal Cluster and Cabin/3(DecelCmd)
  Pedal Cluster Input/2(AccelCmd) -> Pedal Cluster and Cabin/2(AccCmd)
  Pedal Cluster Input/1(SteerCmd) -> Pedal Cluster and Cabin/1(SteerCmd)
  [Driveline] -> Pedal Cluster Input/2(Driveline)
  Pedal Cluster Input/5(BrkPrs) -> Pedal Cluster and Cabin/5(BrkPrs)
  [Steering] -> Pedal Cluster Input/3(Steering)
  Pedal Cluster Input/6(StrWhlTrq) -> Pedal Cluster and Cabin/6(StrWhlTrq)
  "Body, Suspension, Wheels"/2(Wheels) -> Chassis Output/2(Wheels)
  "Body, Suspension, Wheels"/1(Veh) -> Chassis Output/1(Veh)
  Chassis Output/2(WheelsFdbk) -> [Wheels], Out Bus Element5/1
  Chassis Output/1(VehFdbk) -> Out Bus Element4/1
  "Steering, Transmission, Driveline and Brakes"/7(Gear) -> Driveline Output/7(Gear)
  Chassis Input/3(DCM) -> "Body, Suspension, Wheels"/3(DCM)

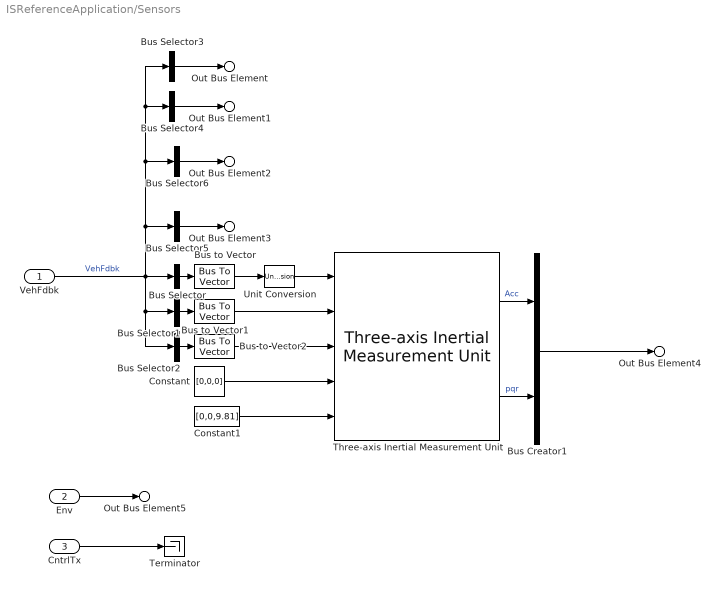
== system ISReferenceApplication/Sensors ==
  VehFdbk : Inport
  Env : Inport  Port=2
  CntrlTx : Inport  Port=3
  Bus Creator1 : BusCreator  Inputs=2
  Bus Selector : BusSelector  OutputSignals=Body.BdyFrm.Cg.Acc.ax,Body.BdyFrm.Cg.Acc.ay,Body.BdyFrm.Cg.Acc.az  OutputAsBus=on
  Bus Selector1 : BusSelector  OutputSignals=Body.BdyFrm.Cg.AngVel.p,Body.BdyFrm.Cg.AngVel.q,Body.BdyFrm.Cg.AngVel.r  OutputAsBus=on
  Bus Selector2 : BusSelector  OutputSignals=Body.BdyFrm.Cg.AngAcc.pdot,Body.BdyFrm.Cg.AngAcc.qdot,Body.BdyFrm.Cg.AngAcc.rdot  OutputAsBus=on
  Bus Selector3 : BusSelector  OutputSignals=Driver  OutputAsBus=on
  Bus Selector4 : BusSelector  OutputSignals=Engine.EngTrq,Driveline.EngSpd  OutputAsBus=on
  Bus Selector5 : BusSelector  OutputSignals=Driveline.BrkPrs,Wheels.TireFrame.Kappa,Wheels.TireFrame.Alpha,Wheels.TireFrame.Omega  OutputAsBus=on
  Bus Selector6 : BusSelector  OutputSignals=Driveline.PropShftSpd,Driveline.AxlTrq  OutputAsBus=on
  Bus to Vector : BusToVector
  Bus to Vector1 : BusToVector
  Bus to Vector2 : BusToVector
  Constant : Constant  Value=[0,0,0]
  Constant1 : Constant  Value=[0,0,9.81]
  Terminator : Terminator
  Three-axis Inertial Measurement Unit : vehdynlibsens/Three-axis Inertial Measurement Unit  units=Metric (MKS)  imu=[0 0 0]  i_Ts=0  dtype_a=off  w_a=190  z_a=0.707  a_sf_cc=[1 0 0; 0 1 0; 0 0 1]  a_bias=[0 0 0]  a_sat="[-inf  -inf  -inf  inf inf inf]"  dtype_g=off  w_g=190  z_g=0.707  g_sf_cc=[1 0 0; 0 1 0; 0 0 1]  g_bias=[0 0 0]  g_sens=[0 0 0]  g_sat="[-inf  -inf  -inf  inf inf inf]"  i_rand=on  i_seeds=[23093 23094 23095 23096 23097 23098]  i_pow=[0.001 0.001 0.001 0.0001 0.0001 0.0001]  aMode=2
  Unit Conversion : UnitConversion
  Out Bus Element : Outport  PortName=CntrlRx  Element=Driver
  Out Bus Element1 : Outport  PortName=CntrlRx  Element=Engine
  Out Bus Element2 : Outport  PortName=CntrlRx  Element=Trans
  Out Bus Element3 : Outport  PortName=CntrlRx  Element=Wheels
  Out Bus Element4 : Outport  PortName=CntrlRx  Element=IMU
  Out Bus Element5 : Outport  PortName=CntrlRx  Element=Env
  wires:
  VehFdbk/1 -> Bus Selector/1, Bus Selector2/1, Bus Selector1/1, Bus Selector6/1, Bus Selector3/1, Bus Selector4/1, Bus Selector5/1  "VehFdbk"
  Bus Creator1/1 -> Out Bus Element4/1
  Three-axis Inertial Measurement Unit/1 -> Bus Creator1/1  "Acc"
  Three-axis Inertial Measurement Unit/2 -> Bus Creator1/2  "pqr"
  Bus Selector/1 -> Bus to Vector/1
  Bus to Vector/1 -> Unit Conversion/1
  Bus Selector1/1 -> Bus to Vector1/1
  Bus to Vector1/1 -> Three-axis Inertial Measurement Unit/2
  Env/1 -> Out Bus Element5/1
  Bus Selector2/1 -> Bus to Vector2/1
  Constant/1 -> Three-axis Inertial Measurement Unit/4
  Unit Conversion/1 -> Three-axis Inertial Measurement Unit/1
  CntrlTx/1 -> Terminator/1
  Bus Selector3/1 -> Out Bus Element/1
  Bus Selector4/1 -> Out Bus Element1/1
  Bus Selector5/1 -> Out Bus Element3/1
  Bus Selector6/1 -> Out Bus Element2/1
  Constant1/1 -> Three-axis Inertial Measurement Unit/5
  Bus to Vector2/1 -> Three-axis Inertial Measurement Unit/3

== system ISReferenceApplication/Subsystem4 ==

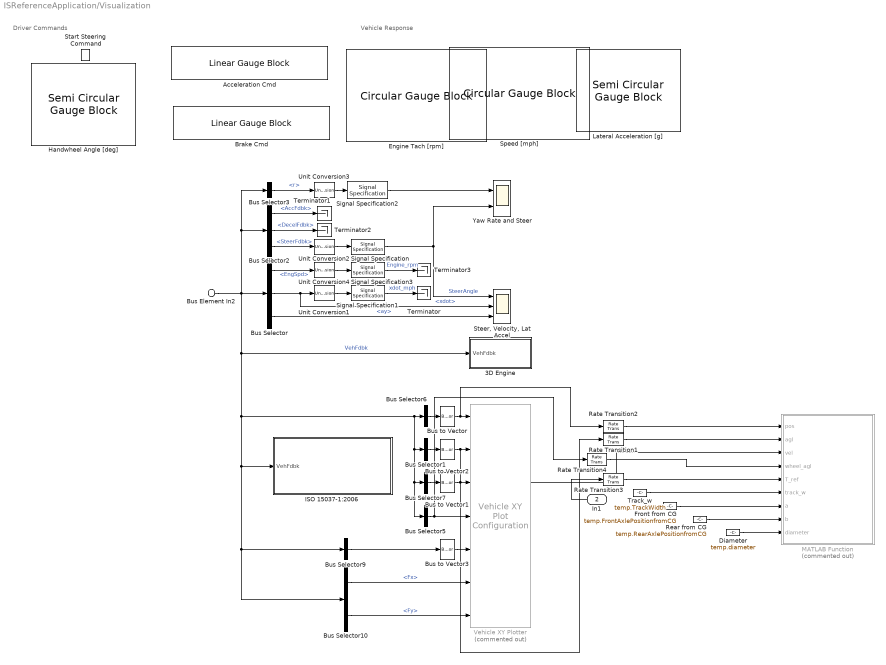
== system ISReferenceApplication/Visualization ==
  note: Driver Commands
  note: Vehicle Response
  Bus Element In2 : Inport  PortName=VehFdbk
  In1 : Inport  Port=2
  3D Engine : Subsystem  Variant=on  mask(3D Engine){engine3D=Disabled, use3DOp=off, SceneDesc=Open surface, dt3D=.05, defaultPos=Recommended for scene, X_o=0, Y_o=0, Z_o=0, phi_o=0, theta_o=0, psi_o=0}
      mask prompts: engine3D "vdynblks:vehdynRefApp3DEng:blkPrm_engine3D"; use3DOp "Use default operating point"; SceneDesc "shared_sim3dblks:sim3dblkConfig:SceneDesc"; dt3D "vdynblks:vehdynRefApp3DEng:blkPrm_dt3D"; X_o "vdynblks:vehdynRefApp3DEng:blkPrm_X_o"; Y_o "vdynblks:vehdynRefApp3DEng:blkPrm_Y_o"; Z_o "vdynblks:vehdynRefApp3DEng:blkPrm_Z_o"; phi_o "vdynblks:vehdynRefApp3DEng:blkPrm_phi_o"; theta_o "vdynblks:vehdynRefApp3DEng:blkPrm_theta_o"; psi_o "vdynblks:vehdynRefApp3DEng:blkPrm_psi_o"
      mask help: This subsystem contains the interface blocks which permit the display of the vehicle in the 3D virtual environment. Enable it to view the simulation progress, disable it to inhibit the display.
      mask init:
      | GrndFdbkPath = find_system(bdroot(gcb), 'MatchFilter', @Simulink.match.allVariants,'BlockType','SubSystem','Name','Ground Feedback');
      | ManBlkName = 'Slowly Increasing Steer';
      | ManBlkPath = find_system(bdroot(gcb), 'MatchFilter', @Simulink.match.allVariants,'BlockType','SubSystem','Name',ManBlkName);
      | OpVarName = 'dlcSS35mph';
      | switch get_param(gcb,'engine3D')    
      |     case 'Disabled'
      |         try
      |             set_param(GrndFdbkPath{:},'OverrideUsingVariant','0');
      |         catch
      |             disp('Warning: No ground feedback sensor not set')
      |         end
      |         try
      |             if strcmp(get_param(gcb,'use3DOp'),'on') && strcmp(get_param(ManBlkPath{:},'ssMode'),'Resume from a workspace variable')
      |                 set_param(ManBlkPath{:},'ssVar',OpVarName);
      |             end
      |         catch
      |              disp('Warning: Maneuver source block not found. Steady state operating point not set')
      |         end
      |     case 'Enabled'
      |         try
      |             set_param(GrndFdbkPath{:},'OverrideUsingVariant','1');            
      |         catch
      |             disp('Warning: Ground feedback from game engine was not found. Using constant values from model instead.')
      |         end
      |         try
      |             if strcmp(get_param(gcb,'use3DOp'),'on') && strcmp(get_param(ManBlkPath{:},'ssMode'),'Resume from a workspace variable')
      |                 set_param(ManBlkPath{:},'ssVar',[OpVarName '3D']);
      |             end
      |         catch
      |              disp('Warning: Maneuver source block not found. Steady state operating point not set')
      |         end
      |     otherwise
      | end
      settings: AttributesFormatString=|
      | %<SceneDesc>
      | %<engine3D>
      mask Help: eval('vdynblkshelp(''vdynblks3dengine'')');
      mask TypeOptions engine3D: vdynblks:vehdynRefApp3DEng:blkRdBt_engine3D_c1 | vdynblks:vehdynRefApp3DEng:blkRdBt_engine3D_c2
      mask Callback engine3D:
      | switch get_param(gcb,'engine3D')
      |     case 'Disabled'
      |         try
      |             % add specifics here if needed
      |         catch
      |             disp('Warning: Maneuver source block not found in model')
      |         end
      |     case 'Enabled'
      |         try
      |             % add specifics here if needed
      |         catch
      |             disp('Warning: Maneuver source block not found in model')
      |         end
      |     otherwise
      | end
      mask TypeOptions SceneDesc: 3D Engine/Simulation 3D Scene Configuration/SceneDesc
      mask Callback SceneDesc:
      | defaultStatus = get_param(gcb,'defaultPos');
      | if strcmp(defaultStatus,'Recommended for scene')
      | sceneType = get_param(gcb,'SceneDesc');
      | switch sceneType
      |     case 'Straight road'
      |         set_param(gcb,'X_o', '-118')
      |         set_param(gcb,'Y_o', '5.7')
      |         set_param(gcb,'Z_o', '0')
      |         set_param(gcb,'phi_o', '0')
      |         set_param(gcb,'theta_o', '0')
      |         set_param(gcb,'psi_o', '0')
      |     case 'Curved road'
      |         set_param(gcb,'X_o', '0.2')
      |         set_param(gcb,'Y_o', '-1605.0')
      |         set_param(gcb,'Z_o', '0')
      |         set_param(gcb,'phi_o', '0')
      |         set_param(gcb,'theta_o', '0')
      |         set_param(gcb,'psi_o', '-156*pi/180')
      |     case 'Parking lot'
      |         set_param(gcb,'X_o', '-104.0')
      |         set_param(gcb,'Y_o', '-9.7')
      |         set_param(gcb,'Z_o', '0')
      |         set_param(gcb,'phi_o', '0')
      |         set_param(gcb,'theta_o', '0')
      |         set_param(gcb,'psi_o', '0')
      |     case 'Double lane change'
      |         set_param(gcb,'X_o', '0')
      |         set_param(gcb,'Y_o', '5.7')
      |         set_param(gcb,'Z_o', '0')
      |         set_param(gcb,'phi_o', '0')
      |         set_param(gcb,'theta_o', '0')
      |         set_param(gcb,'psi_o', '0')
      |     case 'Open surface'
      |         set_param(gcb,'X_o', '0')
      |         set_param(gcb,'Y_o', '0')
      |         set_param(gcb,'Z_o', '0')
      |         set_param(gcb,'phi_o', '0')
      |         set_param(gcb,'theta_o', '0')
      |         set_param(gcb,'psi_o', '0')
      |     case 'US highway'
      |         set_param(gcb,'X_o', '3592.00')
      |         set_param(gcb,'Y_o', '2617.00')
      |         set_param(gcb,'Z_o', '-1.0')
      |         set_param(gcb,'phi_o', '0')
      |         set_param(gcb,'theta_o', '0')
      |         set_param(gcb,'psi_o', '0')
      |     case 'US city block'
      |         set_param(gcb,'X_o', '-125.19')
      |         set_param(gcb,'Y_o', '1.65')
      |         set_param(gcb,'Z_o', '-0.04')
      |         set_param(gcb,'phi_o', '0')
      |         set_param(gcb,'theta_o', '0')
      |         set_param(gcb,'psi_o', '0')
      |     case 'Large parking lot'
      |         set_param(gcb,'X_o', '45.0')
      |         set_param(gcb,'Y_o', '54.7')
      |         set_param(gcb,'Z_o', '0.0')
      |         set_param(gcb,'phi_o', '0')
      |         set_param(gcb,'theta_o', '0')
      |         set_param(gcb,'psi_o', '-pi/2')
      |     case 'Virtual Mcity'
      |         set_param(gcb,'X_o', '-26.0')
      |         set_param(gcb,'Y_o', '76.0')
      |         set_param(gcb,'Z_o', '0.0')
      |         set_param(gcb,'phi_o', '0')
      |         set_param(gcb,'theta_o', '0')
      |         set_param(gcb,'psi_o', '-40*pi/180')
      |    case 'Suburban'
      |         set_param(gcb,'X_o', '60')
      |         set_param(gcb,'Y_o', '-41.7')
      |         set_param(gcb,'Z_o', '0.0')
      |         set_param(gcb,'phi_o', '0')
      |         set_param(gcb,'theta_o', '0')
      |         set_param(gcb,'psi_o', '-0.192')
      |     otherwise
      |         set_param(gcb,'X_o', '0')
      |         set_param(gcb,'Y_o', '0')
      |         set_param(gcb,'Z_o', '0')
      |         set_param(gcb,'phi_o', '0')
      |         set_param(gcb,'theta_o', '0')
      |         set_param(gcb,'psi_o', '0')
      | end
      | end
      mask TypeOptions defaultPos: vdynblks:vehdynRefApp3DEng:blkRdBt_defaultPos_c1 | vdynblks:vehdynRefApp3DEng:blkRdBt_defaultPos_c2
      mask DialogControl engineConfig Prompt: vdynblks:vehdynRefApp3DEng:blkDlg_engineConfig
      mask DialogControl engine3D Prompt: 3D エンジン
      mask DialogControl SceneDesc Prompt: シーン名:
      mask DialogControl dt3D Prompt: 3D エンジンのフレーム レート、dt3D [s]:
      mask DialogControl posSetup Prompt: vdynblks:vehdynRefApp3DEng:blkDlg_posSetup
      mask DialogControl posSetupDesc Prompt: vdynblks:vehdynRefApp3DEng:blkDisTxt_posSetupDesc
      mask DialogControl X_o Prompt: 縦方向の初期位置、X_o [m]:
      mask DialogControl Y_o Prompt: 横方向の初期位置、Y_o [m]:
      mask DialogControl Z_o Prompt: 垂直方向の初期位置、Z_o [m]:
      mask DialogControl phi_o Prompt: 初期ロール角、phi_o [rad]:
      mask DialogControl theta_o Prompt: 初期ピッチ角、theta_o [rad]:
      mask DialogControl psi_o Prompt: 初期ヨー角、psi_o [rad]:
      mask DialogControl setModelPos Prompt: vdynblks:vehdynRefApp3DEng:blkDlg_setModelPos
      mask DialogControl setModelPos Callback:
      | if strcmp(get_param(bdroot(gcb),'SimulationStatus'),'stopped')
      |     sceneType = get_param(gcb,'SceneDesc');
      |     rootModel = bdroot(gcb);
      |     ws = get_param(rootModel, 'modelworkspace');
      |     VEH = getVariable(ws,'VEH');
      |     ParamList={'X_o',[1,1],{};'Y_o',[1,1],{};'Z_o',[1,1],{};'phi_o',[1,1],{'gte',-pi/2;'lte',pi/2};'theta_o',[1,1],{'gte',-pi/2;'lte',pi/2};'psi_o',[1,1],{'gte',-2*pi;'lte',2*pi}};
      |     paramStruct = autoblkscheckparams(gcb, '3D Engine',ParamList);
      |     VEH.InitialLongPosition = paramStruct.X_o;
      |     VEH.InitialLatPosition = paramStruct.Y_o;
      |     VEH.InitialVertPosition = paramStruct.Z_o;
      |     VEH.InitialRollAngle = paramStruct.phi_o;
      |     VEH.InitialPitchAngle = paramStruct.theta_o;
      |     VEH.InitialYawAngle = paramStruct.psi_o;
      |     assignin(ws,'VEH',VEH);
      |     modelList = {'PassVeh14DOF','PassVeh7DOF'};
      |     for idx =1:length(modelList)
      | %         try
      |             load_system(modelList{idx});
      |             ws = get_param(modelList{idx}, 'modelworkspace');
      |             assignin(ws,'VEH',VEH);
      |             save_system(modelList{idx});
      |             close_system(modelList{idx});
      | %         catch
      | %             disp(['Cannot find ' modelList{idx}])
      | %         end
      |     end
      | end
      mask Display: disp('3D Engine')
  Acceleration Cmd : LinearGaugeBlock  LabelPosition=Hide  ScaleMax=1  TickInterval=0.20000000000000001
  Brake Cmd : LinearGaugeBlock  LabelPosition=Hide  ScaleMax=1  TickInterval=0.20000000000000001
  Bus Selector : BusSelector  OutputSignals=Driveline.EngSpd,Body.BdyFrm.Cg.Vel.xdot,Body.BdyFrm.Cg.Acc.ay
  Bus Selector1 : BusSelector  OutputSignals=Body.InertFrm.Cg.Ang.phi,Body.InertFrm.Cg.Ang.theta,Body.InertFrm.Cg.Ang.psi  OutputAsBus=on
  Bus Selector10 : BusSelector  OutputSignals=Wheels.TireFrame.Fx,Wheels.TireFrame.Fy
  Bus Selector2 : BusSelector  OutputSignals=Driver.AccFdbk,Driver.DecelFdbk,Driver.SteerFdbk
  Bus Selector3 : BusSelector  OutputSignals=Body.BdyFrm.Cg.AngVel.r
  Bus Selector5 : BusSelector  OutputSignals=Driveline.WhlAng  OutputAsBus=on
  Bus Selector6 : BusSelector  OutputSignals=Body.InertFrm.Geom.Disp.X,Body.InertFrm.Geom.Disp.Y,Body.InertFrm.Geom.Disp.Z  OutputAsBus=on
  Bus Selector7 : BusSelector  OutputSignals=Body.InertFrm.Geom.Vel.Xdot,Body.InertFrm.Geom.Vel.Ydot,Body.InertFrm.Geom.Vel.Zdot  OutputAsBus=on
  Bus Selector9 : BusSelector  OutputSignals=Driveline.EngSpd,Driveline.Gear  OutputAsBus=on
  Bus to Vector{,1..3} (4 alike) : BusToVector
  Diameter : Constant  Value=temp.diameter
  Engine Tach [rpm] : CircularGaugeBlock  LabelPosition=Hide  ScaleMax=8000  TickInterval=1000
  Front from CG : Constant  Value=temp.FrontAxlePositionfromCG
  Handwheel Angle [deg] : SemiCircularGaugeBlock  LabelPosition=Hide  ScaleMin=-300  ScaleMax=300  TickInterval=60
  ISO 15037-1:2006 : Subsystem  StopFcn=|  Variant=on  VariantControlMode=label  LabelModeActiveChoice=0  mask(ISO 15037-1:2006){Measurement=Disabled}
      | switch get_param(gcb,'Measurement')
      |     case 'Enabled'
      |        p=slproject.getCurrentProject;
      |        projectRoot=p.RootFolder;
      |        SySFolder=fullfile(projectRoot, 'System');
      |        Simulink.sdi.loadView([SySFolder filesep 'ISO15037_1_2006E.mldatx']);
      |        Simulink.sdi.view;
      | end
      mask prompts: Measurement "ISO Measurements"
      mask help: Enables display of ISO 15037-1:2006 standard measurement signals in the Simulation Data Inspector.
      mask init:
      | switch get_param(gcb,'Measurement')
      |     case 'Disabled'
      |         set_param(gcb,'OverrideUsingVariant','0')
      |     case 'Enabled'
      |        set_param(gcb,'OverrideUsingVariant','1')
      |     otherwise
      |        set_param(gcb,'OverrideUsingVariant','0')
      | end
      settings: AttributesFormatString=%<Measurement>
      mask Help: eval('vdynblkshelp(''iso15037'')');
      mask TypeOptions Measurement: Enabled | Disabled
      mask Callback Measurement:
      | switch get_param(gcb,'Measurement')
      |     case 'Disabled'
      |         set_param(gcb,'OverrideUsingVariant','0')
      |     case 'Enabled'
      |        set_param(gcb,'OverrideUsingVariant','1')
      |     otherwise
      |        set_param(gcb,'OverrideUsingVariant','0')
      | end
      mask Display: disp('ISO 15037-1:2006')
  Lateral Acceleration [g] : SemiCircularGaugeBlock  LabelPosition=Hide  ScaleMin=-1  ScaleMax=1  TickInterval=0.5
  MATLAB Function : MATLAB Function  Commented=on  TreatAsAtomicUnit=on
  Rate Transition{1..4} (4 alike) : RateTransition  Deterministic=off  OutPortSampleTime=temp.DrawFreq
  Rear from CG : Constant  Value=temp.RearAxlePositionfromCG
  Signal Specification : SignalSpecification  Unit=deg
  Signal Specification1 : SignalSpecification  Unit=mph
  Signal Specification2 : SignalSpecification  Unit=deg/s
  Signal Specification3 : SignalSpecification  Unit=rpm
  Speed [mph] : CircularGaugeBlock  LabelPosition=Hide  TickInterval=10
  Start Steering Command : LampBlock  LabelPosition=Hide
  "Steer, Velocity, Lat Accel" : Scope  NumInputPorts=3
  Terminator{,1..3} (4 alike) : Terminator
  Track_w : Constant  Value=temp.TrackWidth
  Unit Conversion{1..4} (4 alike) : UnitConversion
  Vehicle XY Plotter : vehdynlibviscommon/Vehicle XY Plot Configuration  Commented=on  extRef=off  extStats=on  extTireF=on  a=temp.FrontAxlePositionfromCG  b=temp.RearAxlePositionfromCG  w=temp.TrackWidth  figBorder=10  bufferSize=1024  velNorm=5  tireFNorm=1000  pltDT=.1
  Yaw Rate and Steer : Scope  NumInputPorts=2
  wires:
  Unit Conversion3/1 -> Signal Specification2/1
  Bus Selector3/1 -> Unit Conversion3/1  "<r>"
  Signal Specification2/1 -> Yaw Rate and Steer/1
  Bus to Vector3/1 -> Vehicle XY Plotter/5
  Bus Selector/3 -> "Steer, Velocity, Lat Accel"/3  "<ay>"
  Signal Specification3/1 -> Terminator3/1  "Engine_rpm"
  Bus Selector9/1 -> Bus to Vector3/1
  Bus Element In2/1 -> Bus Selector10/1, Bus Selector9/1, ISO 15037-1:2006/1(VehFdbk), Bus Selector5/1, Bus Selector7/1, Bus Selector1/1, Bus Selector6/1, 3D Engine/1(VehFdbk), Bus Selector3/1, Bus Selector2/1, Bus Selector/1  "VehFdbk"
  Bus Selector2/2 -> Terminator2/1  "<DecelFdbk>"
  Bus to Vector2/1 -> Rate Transition1/1, Vehicle XY Plotter/2
  Bus Selector6/1 -> Bus to Vector/1
  Bus to Vector/1 -> Rate Transition2/1, Vehicle XY Plotter/1
  Bus Selector1/1 -> Bus to Vector2/1
  Bus to Vector1/1 -> MATLAB Function/3(vel), Vehicle XY Plotter/3
  Bus Selector7/1 -> Bus to Vector1/1
  Unit Conversion4/1 -> Signal Specification3/1
  Bus Selector/1 -> Unit Conversion4/1  "<EngSpd>"
  Bus Selector2/1 -> Terminator1/1  "<AccFdbk>"
  Bus Selector2/3 -> Unit Conversion2/1  "<SteerFdbk>"
  Bus Selector10/2 -> Vehicle XY Plotter/7  "<Fy>"
  Signal Specification1/1 -> Terminator/1  "xdot_mph"
  Unit Conversion1/1 -> Signal Specification1/1
  Signal Specification/1 -> Yaw Rate and Steer/2, "Steer, Velocity, Lat Accel"/1  "SteerAngle"
  Bus Selector10/1 -> Vehicle XY Plotter/6  "<Fx>"
  Unit Conversion2/1 -> Signal Specification/1
  Bus Selector/2 -> "Steer, Velocity, Lat Accel"/2, Unit Conversion1/1  "<xdot>"
  Bus Selector5/1 -> Vehicle XY Plotter/4, Rate Transition4/1
  Rate Transition4/1 -> MATLAB Function/4(wheel_agl)
  Rate Transition1/1 -> MATLAB Function/2(agl)
  Rate Transition2/1 -> MATLAB Function/1(pos)
  In1/1 -> Rate Transition3/1
  Rate Transition3/1 -> MATLAB Function/5(T_ref)
  Track_w/1 -> MATLAB Function/6(track_w)
  Front from CG/1 -> MATLAB Function/7(a)
  Rear from CG/1 -> MATLAB Function/8(b)
  Diameter/1 -> MATLAB Function/9(diameter)

== system ISReferenceApplication/Controllers/Active Differential Control ==
  note: 1) Add Subsystem or Model blocks as valid variant choices.
      | 2) You cannot connect blocks at this level. At simulation, connectivity is automatically
      | determined, based on the active variant and port name matching.
  Accel : Inport
  BrkCmd : Inport  Port=2
  Steer : Inport  Port=3
  GearFdbk : Inport  Port=4
  Omega : Inport  Port=5  Unit=rad/s
  axayaz : Inport  Port=6
  pqr : Inport  Port=7
  No Control : Subsystem  VariantControl=0
  Rear Diff Controller : Subsystem  TreatAsAtomicUnit=on  SystemSampleTime=.01  VariantControl=1
  DiffPrsCmd : Outport  VectorParamsAs1DForOutWhenUnconnected=off
  TrqCmd : Outport  Port=2  VectorParamsAs1DForOutWhenUnconnected=off

== system ISReferenceApplication/Controllers/Brake Pressure Control ==
  note: 1) Add Subsystem or Model blocks as valid variant choices.
      | 2) You cannot connect blocks at this level. At simulation, connectivity is automatically
      | determined, based on the active variant and port name matching.
  DecelFdbk : Inport
  Omega : Inport  Port=2
  Accel : Inport  Port=3
  AccelFdbk : Inport  Port=4
  BrkPrs : Inport  Port=5
  Bang Bang ABS : Subsystem  VariantControl=1
  Five-State ABS and TCS : Subsystem  VariantControl=2
  Open Loop : Subsystem  VariantControl=0
  ABSFlag : Outport  VectorParamsAs1DForOutWhenUnconnected=off
  BrkPrsCmd : Outport  Port=2  VectorParamsAs1DForOutWhenUnconnected=off
  TCSFlag : Outport  Port=3  VectorParamsAs1DForOutWhenUnconnected=off

== system ISReferenceApplication/Controllers/ECU ==
  DiffTrqCmd : Inport
  <Accel> : Inport  Port=2
  EngSpd : Inport  Port=3
  ABSFlag : Inport  Port=4
  First Order Hold : FirstOrderHold  ErrorTolerance=100
  Torque Cmd : Subsystem  TreatAsAtomicUnit=on  SystemSampleTime=.01
  EngTrqCmd : Outport  VectorParamsAs1DForOutWhenUnconnected=off
  wires:
  First Order Hold/1 -> EngTrqCmd/1
  DiffTrqCmd/1 -> Torque Cmd/1(DiffTrqCmd)
  <Accel>/1 -> Torque Cmd/2(<Accel>)
  EngSpd/1 -> Torque Cmd/3(EngSpd)
  Torque Cmd/1(EngTrqCmd) -> First Order Hold/1
  ABSFlag/1 -> Torque Cmd/4(ABSFlag)

== system ISReferenceApplication/Controllers/Transmission Controller ==
  Accel : Inport
  BrkCmd : Inport  Port=2
  GearReq : Inport  Port=3
  EngSpd : Inport  Port=4
  Omega : Inport  Port=5  Unit=rad/s
  ABSFlag : Inport  Port=6
  UpReq : Inport  Port=7
  DownReq : Inport  Port=8  Unit=rad/s
  Driver - No Clutch : Subsystem  VariantControl=1
  PRNDL Controller : Subsystem  VariantControl=3
  Paddles : Subsystem  VariantControl=2
  Transmission Controller : Subsystem  VariantControl=0
  " Gear" : Outport  VectorParamsAs1DForOutWhenUnconnected=off

== system ISReferenceApplication/Driver Commands/Driver Commands ==
  VehRef : Inport
  VehFdbk : Inport  Port=2
  SteerCmd : Inport  Port=3
  AccelCmd : Inport  Port=4
  BrakeCmd : Inport  Port=5
  GearCmd : Inport  Port=6
  Longitudinal Driver : Subsystem  VariantControl=driverType==1
  Open Loop : Subsystem  VariantControl=driverType==3
  Predictive Driver : Subsystem  VariantControl=driverType==2
  " Driver" : Outport  VectorParamsAs1DForOutWhenUnconnected=off
